simulink model "fetft_preisach_write_hold_read"  (R2026a)
settings: Solver=FixedStepDiscrete  StopTime=4e-05  FixedStep=5e-08
InitFcn:
  | preisachSequenceInput = fetft_preisach_sequence_dataset;
settings Model: Creator=elesamj  LastModifiedBy=elesamj

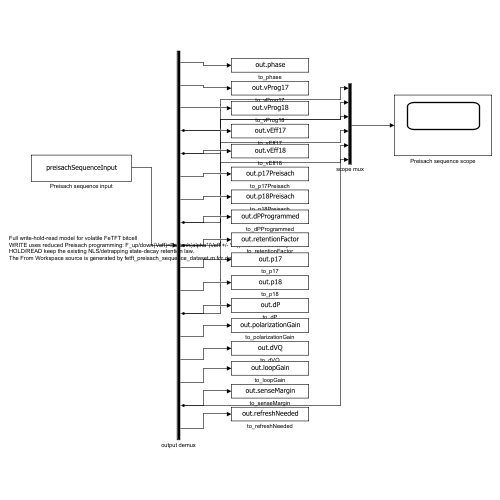
[thumbnail: Simulink's stored preview of the top-level diagram]
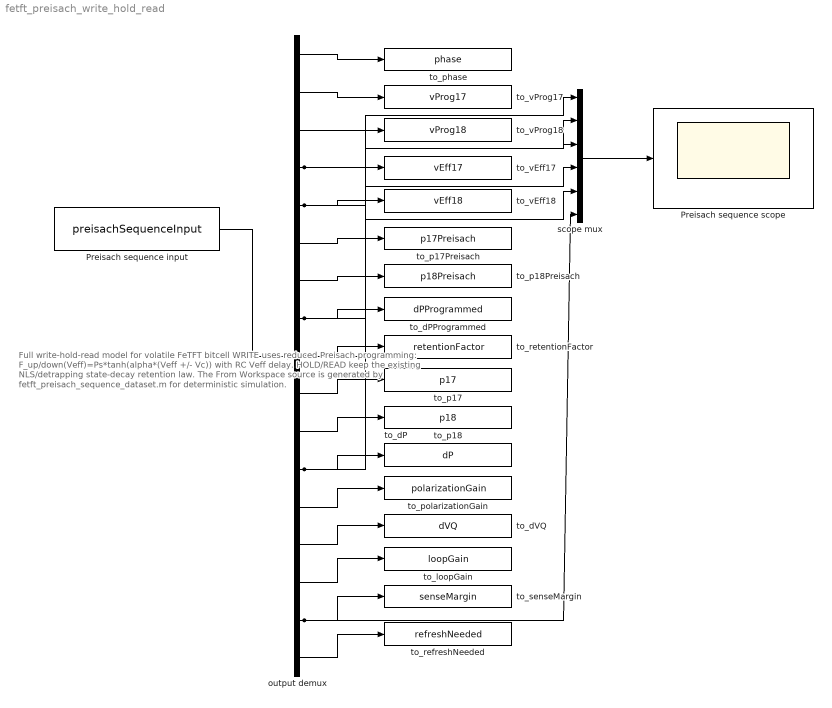
== system fetft_preisach_write_hold_read ==
  note: Full write-hold-read model for volatile FeTFT bitcell
      | WRITE uses reduced Preisach programming: F_up/down(Veff)=Ps*tanh(alpha*(Veff +/- Vc)) with RC Veff delay.
      | HOLD/READ keep the existing NLS/detrapping state-decay retention law.
      | The From Workspace source is generated by fetft_preisach_sequence_dataset.m for deterministic simulation.
  Preisach sequence input : FromWorkspace  VariableName=preisachSequenceInput  Interpolate=off  OutputAfterFinalValue=Holding final value
  Preisach sequence scope : Scope
  output demux : Demux  Outputs=17
  scope mux : Mux  Inputs=6
  to_dP : ToWorkspace  VariableName=dP  SaveFormat=Structure With Time  SampleTime=-1
  to_dPProgrammed : ToWorkspace  VariableName=dPProgrammed  SaveFormat=Structure With Time  SampleTime=-1
  to_dVQ : ToWorkspace  VariableName=dVQ  SaveFormat=Structure With Time  SampleTime=-1
  to_loopGain : ToWorkspace  VariableName=loopGain  SaveFormat=Structure With Time  SampleTime=-1
  to_p17 : ToWorkspace  VariableName=p17  SaveFormat=Structure With Time  SampleTime=-1
  to_p17Preisach : ToWorkspace  VariableName=p17Preisach  SaveFormat=Structure With Time  SampleTime=-1
  to_p18 : ToWorkspace  VariableName=p18  SaveFormat=Structure With Time  SampleTime=-1
  to_p18Preisach : ToWorkspace  VariableName=p18Preisach  SaveFormat=Structure With Time  SampleTime=-1
  to_phase : ToWorkspace  VariableName=phase  SaveFormat=Structure With Time  SampleTime=-1
  to_polarizationGain : ToWorkspace  VariableName=polarizationGain  SaveFormat=Structure With Time  SampleTime=-1
  to_refreshNeeded : ToWorkspace  VariableName=refreshNeeded  SaveFormat=Structure With Time  SampleTime=-1
  to_retentionFactor : ToWorkspace  VariableName=retentionFactor  SaveFormat=Structure With Time  SampleTime=-1
  to_senseMargin : ToWorkspace  VariableName=senseMargin  SaveFormat=Structure With Time  SampleTime=-1
  to_vEff17 : ToWorkspace  VariableName=vEff17  SaveFormat=Structure With Time  SampleTime=-1
  to_vEff18 : ToWorkspace  VariableName=vEff18  SaveFormat=Structure With Time  SampleTime=-1
  to_vProg17 : ToWorkspace  VariableName=vProg17  SaveFormat=Structure With Time  SampleTime=-1
  to_vProg18 : ToWorkspace  VariableName=vProg18  SaveFormat=Structure With Time  SampleTime=-1
  wires:
  output demux/1 -> to_phase/1
  output demux/2 -> to_vProg17/1
  output demux/3 -> to_vProg18/1
  output demux/4 -> to_vEff17/1, scope mux/1
  output demux/5 -> to_vEff18/1, scope mux/2
  output demux/6 -> to_p17Preisach/1
  output demux/7 -> to_p18Preisach/1
  output demux/8 -> to_dPProgrammed/1, scope mux/3
  output demux/9 -> to_retentionFactor/1, scope mux/4
  output demux/10 -> to_p17/1
  output demux/11 -> to_p18/1
  output demux/12 -> to_dP/1, scope mux/5
  output demux/13 -> to_polarizationGain/1
  output demux/14 -> to_dVQ/1
  output demux/15 -> to_loopGain/1
  output demux/16 -> to_senseMargin/1, scope mux/6
  output demux/17 -> to_refreshNeeded/1
  Preisach sequence input/1 -> output demux/1
  scope mux/1 -> Preisach sequence scope/1
